simulink subsystem "integrador_discreto"  (R2023b)
settings: Solver=VariableStepAuto  StartTime=0.0  StopTime=10.0  RelTol=1e-3
undefined symbols (not defined in the file or in its folder): T_s
settings Model: Creator=nicol  LastModifiedBy=nicol

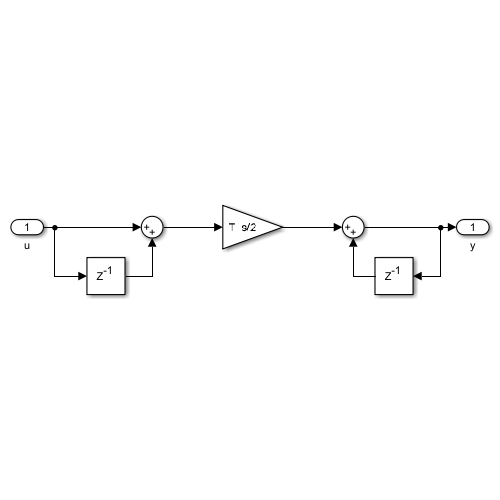
[thumbnail: Simulink's stored preview of the top-level diagram]
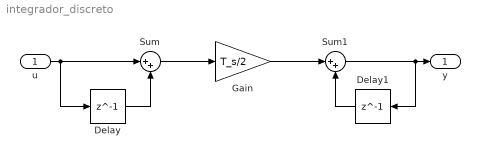
== system integrador_discreto ==
  u : Inport
  Delay : Delay  DelayLength=1  InitialCondition=0
  Delay1 : Delay  DelayLength=1  InitialCondition=0
  Gain : Gain  Gain=T_s/2
  Sum : Sum  Inputs=|++
  Sum1 : Sum  Inputs=|++
  y : Outport
  wires:
  u/1 -> Delay/1, Sum/1
  Delay/1 -> Sum/2
  Sum/1 -> Gain/1
  Gain/1 -> Sum1/1
  Delay1/1 -> Sum1/2
  Sum1/1 -> Delay1/1, y/1
